simulink model "qpsk_coded"  (R2022a)
settings: Solver=VariableStepDiscrete  StartTime=0.0  StopTime=inf  RelTol=1e-3  EnableMultiTasking=on
StopFcn:
  | if BER(1)==0
  | BER(1)=1/BER(3);
  | end
values from neighbouring files (symbols this model uses):
  EbNo = 3.3    [errPattern.m]    (also in symuluj_przeplot.m = 0:0.1:2.9)
libraries: commcnvcod2 x2, commdigbbndpm3 x2, commchan3 x1, commrandsrc2 x1, commsink2 x1
settings Model: Creator=Administrator  LastModifiedBy=User
settings SolverCC: AlgebraicLoopSolver=TrustRegion
settings DataIOCC: LimitDataPoints=on  SaveFormat=Array  SignalLoggingSaveFormat=ModelDataLogs  ReturnWorkspaceOutputs=off
settings OptimizationCC: ExpressionDepthLimit=2147483647  InitFltsAndDblsToZero=on  LifeSpan=inf
settings DebuggingCC: UnderspecifiedInitializationDetection=Classic  MergeDetectMultiDrivingBlocksExec=none  SolverPrmCheckMsg=warning  FcnCallInpInsideContextMsg=warning  UnconnectedInputMsg=warning  UnconnectedOutputMsg=warning  UnconnectedLineMsg=warning  StateNameClashWarn=warning  SFUnexpectedBacktrackingDiag=warning  SFNoUnconditionalDefaultTransitionDiag=warning  SFMachineParentedDataDiag=warning  ArithmeticOperatorsInVariantConditions=warning
settings HardwareCC: ProdBitPerPointer=32  ProdBitPerSizeT=32  ProdBitPerPtrDiffT=32  ProdLargestAtomicFloat=None  ProdIntDivRoundTo=Undefined  ProdEndianess=Unspecified  ProdWordSize=32  ProdHWDeviceType=32-bit Generic
settings ModelReferenceCC: PropagateSignalLabelsOutOfModel=off
settings SFSimCC: SimUseLocalCustomCode=off  CustomCodeUndefinedFunction=UseInterfaceOnly
settings RTWCC: RTWUseLocalCustomCode=off
settings CodeAppCC: StateflowObjectComments=on
settings GRTTargetCC: TargetLangStandard=C89/C90 (ANSI)  CombineOutputUpdateFcns=off  GRTInterface=on
settings ConfigComp: CovMetricSettings=dw  CovSaveCumulativeToWorkspaceVar=on  CovSaveSingleToWorkspaceVar=on  CovExternalEMLEnable=off

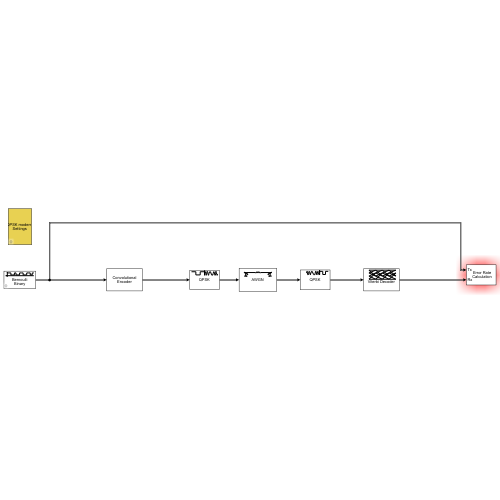
[thumbnail: Simulink's stored preview of the top-level diagram]
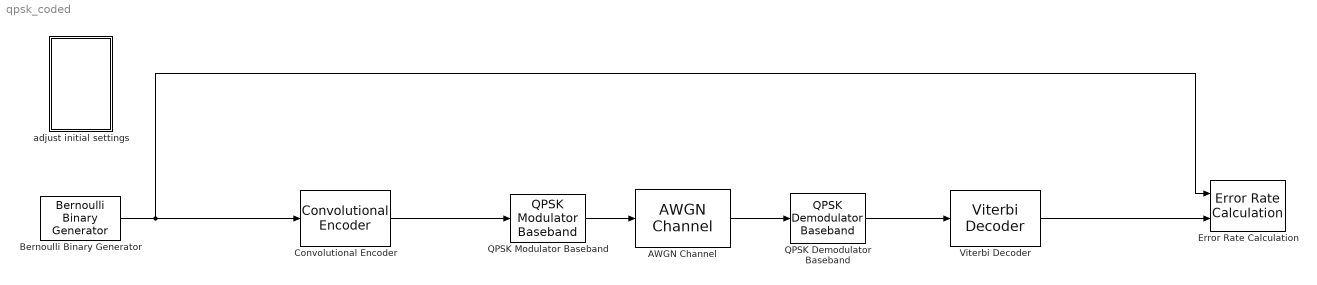
== system qpsk_coded ==
  AWGN Channel : commchan3/AWGN Channel  InputProcessing=Columns as channels (frame based)  seed=67  noiseMode="Signal to noise ratio  (SNR)"  EbNodB=EbNo  EsNodB=10  SNRdB=EbNo + 1.76091  bitsPerSym=2.0  Ps=1  Tsym=1.51515  variance=1
  Bernoulli Binary Generator : commrandsrc2/Bernoulli Binary Generator  P=0.5  seed=61  Ts=1  frameBased=on  sampPerFrame=188*1000*3  orient=off  outDataType=boolean
      settings: SourceProductBaseCode=CM
  Convolutional Encoder : commcnvcod2/Convolutional Encoder  trellis=poly2trellis(7, [171 133])  opMode=Continuous  DelayedResetAction=off  hasIniStPort=off  hasFinStPort=off  usePuncVector=on  punctureVector=[1; 1; 0; 1; 1; 0]  reset=Unused parameter value
      settings: SourceProductBaseCode=CM
  Error Rate Calculation : commsink2/Error Rate Calculation  N=136  st_delay=0  cp_mode=Entire frame  subframe=[]  PMode=Workspace  WsName=BER  RsMode2=off  stop=on  numErr=maxNumErrs  maxBits=maxNumBits
  QPSK Demodulator Baseband : commdigbbndpm3/QPSK Demodulator Baseband  OutType=Bit  DecType=Hard decision  VarSource=Dialog  Variance=(1.0/(2*0.75))*10^(-EbNo/10)  Dec=Gray  Ph=pi/4  outDtype1=boolean  outDtype2=Inherit via internal rule  derotateFactorWordLen=16  derotateFactorDataTypeStr=Inherit: Same word length as input  derotateFactorLastDataTypeStr=Inherit: Same word length as input
  QPSK Modulator Baseband : commdigbbndpm3/QPSK Modulator Baseband  InType=Bit  Enc=Gray  Ph=pi/4  outDtype=double  outWordLen=16  outUDDataType=sfix(16)  outFracLenMode=Best precision  outFracLen=15  outDataTypeStr=double  outLastDataTypeStr=double
  Viterbi Decoder : commcnvcod2/Viterbi Decoder  trellis=poly2trellis(7, [171 133])  isPunctured=on  punctureVector=[1; 1; 0; 1; 1; 0]  erasures=off  dectype=Hard decision  nsdecb=4  runSigValErrCheck=off  tbdepth=136  opmode=Continuous  reset=off  delayedResetAction=off  smWordLength=16  outDataType=boolean
      settings: SourceProductBaseCode=CM
  adjust initial settings : Subsystem  mask(RF Link Demo:Initial Settings){DecType='hard', CodeRate=3/4}
      mask prompts: DecType "Decision type:"; CodeRate "FEC code rate:"
      mask help: Select the scenarios from the mask to change the link parameters. Each of the mask parameters sets the parameters in the corresponding RF impairment block(s).
      mask init:
      | switch CodeRate
      |         case 1, %1/2
      |         codeRate=0.5;
      |         set_param('qpsk_coded/Convolutional Encoder','usePuncVector','off')
      |         set_param('qpsk_coded/Viterbi Decoder','isPunctured','off')
      |         %%set_param('qpsk_coded/AWGN Channel','Tsym','1')
      |         set_param('qpsk_coded/AWGN Channel','SNRdB',sprintf('EbNo + %g',10*log10(2.0*codeRate)))
      |         set_param('qpsk_coded/Bernoulli Binary Generator','sampPerFrame','188*1000')
      | 
      |         case 2, %2/3
      |         codeRate=0.66;
      |         set_param('qpsk_coded/Convolutional Encoder','usePuncVector','on')
      |         set_param('qpsk_coded/Convolutional Encoder','punctureVector','[1; 1; 0; 1]')
      |         set_param('qpsk_coded/Viterbi Decoder','isPunctured','on')
      |         set_param('qpsk_coded/Viterbi Decoder','punctureVector','[1; 1; 0; 1]')
      |         %%set_param('qpsk_coded/AWGN Channel','Tsym','1.334')
      |         set_param('qpsk_coded/AWGN Channel','SNRdB',sprintf('EbNo + %g',10*log10(2.0*codeRate)))        
      |         set_param('qpsk_coded/Bernoulli Binary Generator','sampPerFrame','188*1000')
      | 
      |         case 3, %3/4
      |         codeRate=0.75;
      |         set_param('qpsk_coded/Convolutional Encoder','usePuncVector','on')
      |         set_param('qpsk_coded/Convolutional Encoder','punctureVector','[1; 1; 0; 1; 1; 0]')
      |         set_param('qpsk_coded/Viterbi Decoder','isPunctured','on')
      |         set_param('qpsk_coded/Viterbi Decoder','punctureVector','[1; 1; 0; 1; 1; 0]')
      |         %%set_param('qpsk_coded/AWGN Channel','Tsym','1.5')
      |         set_param('qpsk_coded/AWGN Channel','SNRdB',sprintf('EbNo + %g',10*log10(2.0*codeRate)))        
      |         set_param('qpsk_coded/Bernoulli Binary Generator','sampPerFrame','188*1000*3')
      |         case 4, %5/6
      |         codeRate=0.83;            
      |         set_param('qpsk_coded/Convolutional Encoder','usePuncVector','on')
      |         set_param('qpsk_coded/Convolutional Encoder','punctureVector','[1; 1; 0; 1; 1; 0; 0; 1;1;0]')
      |         set_param('qpsk_coded/Viterbi Decoder','isPunctured','on')
      |         set_param('qpsk_coded/Viterbi Decoder','punctureVector','[1; 1; 0; 1; 1; 0; 0; 1;1;0]')
      |         %%set_param('qpsk_coded/AWGN Channel','Tsym','1.66667')
      |         set_param('qpsk_coded/AWGN Channel','SNRdB',sprintf('EbNo + %g',10*log10(2.0*codeRate)))        
      |         set_param('qpsk_coded/Bernoulli Binary Generator','sampPerFrame','188*5*1000')
      |         case 5, %7/8
      |         codeRate=0.875;            
      |         set_param('qpsk_coded/Convolutional Encoder','usePuncVector','on')
      |         set_param('qpsk_coded/Convolutional Encoder','punctureVector','[1;1;0;1;0;1;0;1;1;0;0;1;1;0]')
      |         set_param('qpsk_coded/Viterbi Decoder','isPunctured','on')
      |         set_param('qpsk_coded/Viterbi Decoder','punctureVector','[1;1;0;1;0;1;0;1;1;0;0;1;1;0]')
      |         %%set_param('qpsk_coded/AWGN Channel','Tsym','1.75')
      |         set_param('qpsk_coded/AWGN Channel','SNRdB',sprintf('EbNo + %g',10*log10(2.0*codeRate)))                
      |         set_param('qpsk_coded/Bernoulli Binary Generator','sampPerFrame','188*7*1000')
      |    end
      | 
      |    switch DecType
      |        case 'hard',
      |            set_param('qpsk_coded/QPSK Demodulator Baseband','DecType','Hard decision')           
      |            set_param('qpsk_coded/Viterbi Decoder','dectype','Hard decision')
      |        case 'soft',
      |            set_param('qpsk_coded/QPSK Demodulator Baseband','DecType','Approximate log-likelihood ratio')                      
      |            set_param('qpsk_coded/QPSK Demodulator Baseband','Variance',sprintf('(1.0/(2*%g))*10^(-EbNo/10)',codeRate))           
      |            set_param('qpsk_coded/Viterbi Decoder','dectype','Unquantized')           
      |    end
      mask TypeOptions DecType: 'hard' | 'soft'
      mask TypeOptions CodeRate: 1/2 | 2/3 | 3/4 | 5/6 | 7/8
      mask Display: disp('QPSK modem:\nSettings');
  wires:
  Bernoulli Binary Generator/1 -> Error Rate Calculation/1, Convolutional Encoder/1
  QPSK Modulator Baseband/1 -> AWGN Channel/1
  AWGN Channel/1 -> QPSK Demodulator Baseband/1
  QPSK Demodulator Baseband/1 -> Viterbi Decoder/1
  Viterbi Decoder/1 -> Error Rate Calculation/2
  Convolutional Encoder/1 -> QPSK Modulator Baseband/1

== system qpsk_coded/adjust initial settings ==
